simulink model "RL_env"  (R2021b)
settings: Solver=FixedStepAuto  StartTime=0.0  StopTime=Inf  FixedStep=info_.slx_sample_time  RelTol=1e-3
values from neighbouring files (symbols this model uses):
  agent_act_number = 2    [RL_menage.m]
  agent_obs_number = 6    [RL_menage.m]
  agent_sample_time_agent = slx_sample_time    (= 0.1)    [RL_menage.m]
  info_ = info_.add(params_to_save,params_to_save_vals)    [RL_menage.m]
  slx_if_input_normalization = 1    [RL_menage.m]
  slx_if_not_constrain = true    [RL_menage.m]
  slx_multiplier = 1    [RL_menage.m]
  slx_ObsMaximal = repmat(slx_ObsMaximal,1,slx_how_many_steps_in_run)    [RL_menage.m]
  slx_ObsMinimal = zeros(agent_obs_number,1); end    [RL_menage.m]
  slx_sample_time = slx_sample_time_in    (= 0.1)    [RL_menage.m]
  slx_use_external = false    [RL_menage.m]
  slx_w1 = slx_w1_in    (= 1)    [RL_menage.m]
  slx_w2 = slx_w2_in    (= 0)    [RL_menage.m]
undefined symbols (not defined in the file or in its folder): agent_data_random_seed_1, agent_data_random_seed_2, slx_constr_bound, umax
libraries: dspindex x2, rllib x1, simulink x1
settings Model: Creator=krzysztof  LastModifiedBy=Randomowa Nazwa
settings DataIOCC: SignalLogging=off
settings ModelReferenceCC: ModelReferenceNumInstancesAllowed=Single

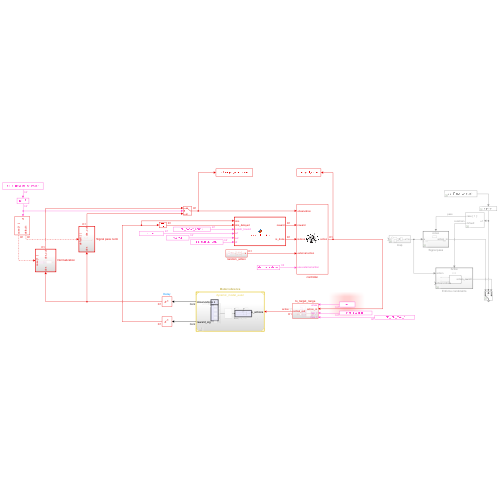
[thumbnail: Simulink's stored preview of the top-level diagram]
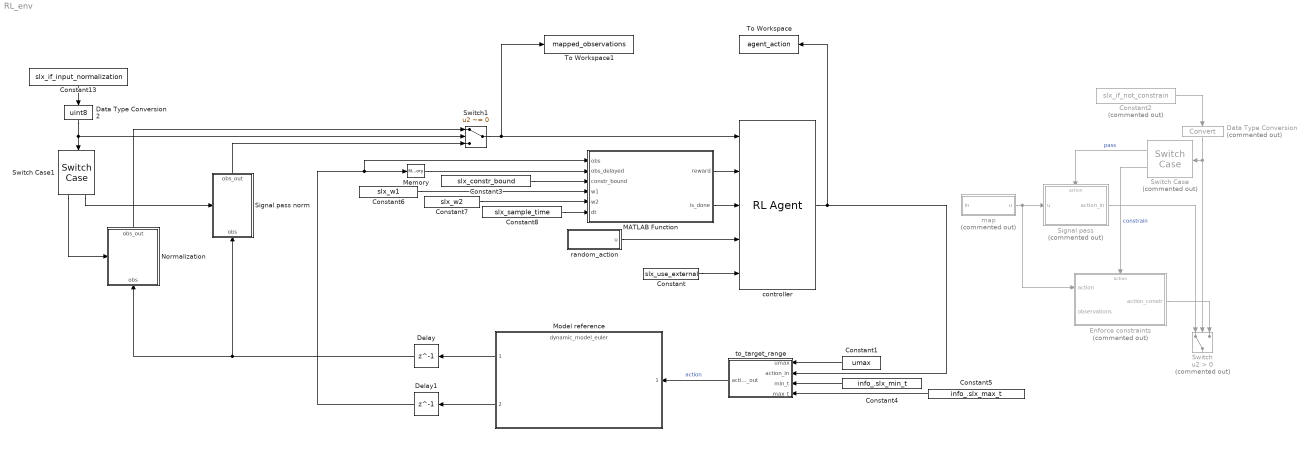
== system RL_env ==
  Constant : Constant  Value=slx_use_external
  Constant1 : Constant  Value=umax
  Constant13 : Constant  Value=slx_if_input_normalization
  Constant2 : Constant  Commented=on  Value=slx_if_not_constrain
  Constant3 : Constant  Value=slx_constr_bound
  Constant4 : Constant  Value=info_.slx_min_t
  Constant5 : Constant  Value=info_.slx_max_t
  Constant6 : Constant  Value=slx_w1
  Constant7 : Constant  Value=slx_w2
  Constant8 : Constant  Value=slx_sample_time
  Data Type Conversion : DataTypeConversion  Commented=on
  Data Type Conversion2 : DataTypeConversion  OutDataTypeStr=uint8
  Delay : Delay  DelayLength=1  InitialCondition=0
  Delay1 : Delay  DelayLength=1  InitialCondition=0
  Enforce constraints : Subsystem  Commented=on  TreatAsAtomicUnit=on
  MATLAB Function : MATLAB Function  TreatAsAtomicUnit=on
  Memory : Memory
  Model reference : ModelReference  ModelNameDialog=dynamic_model_euler.slx  SimulationMode=Normal  ModelReferenceVersion=6.750
  Normalization : Subsystem  TreatAsAtomicUnit=on
  Signal pass : Subsystem  Commented=on  TreatAsAtomicUnit=on
  Signal pass norm : Subsystem  TreatAsAtomicUnit=on
  Switch : Switch  Commented=on  Criteria=u2 > Threshold
  Switch Case : SwitchCase  Commented=on
  Switch Case1 : SwitchCase
  Switch1 : Switch  Criteria=u2 ~= 0
  To Workspace : ToWorkspace  VariableName=agent_action  SaveFormat=Timeseries  SampleTime=-1
  To Workspace1 : ToWorkspace  VariableName=mapped_observations  SaveFormat=Timeseries  SampleTime=-1
  controller : rllib/RL Agent  Agent=agentObj  ExternalActionAsInput=on  ProvideCumRwd=off  TreatAsDirectFeedthrough=on
  map : Subsystem  Commented=on
  random_action : Subsystem
  to_target_range : Subsystem
  wires:
  MATLAB Function/1(reward) -> controller/2
  MATLAB Function/2(is_done) -> controller/3
  Constant/1 -> controller/5
  Constant1/1 -> to_target_range/1(umax)
  Switch Case/2 -> Enforce constraints/Action  "constrain"
  Switch Case/1 -> Signal pass/Action  "pass"
  Signal pass/1(action_in) -> Switch/1
  Enforce constraints/1(action_constr) -> Switch/3
  Constant2/1 -> Data Type Conversion/1
  Data Type Conversion/1 -> Switch/2, Switch Case/1
  Constant3/1 -> MATLAB Function/3(constr_bound)
  random_action/1(u) -> controller/4
  controller/1 -> to_target_range/2(action_in), To Workspace/1
  map/1(u) -> Enforce constraints/1(action), Signal pass/1(u)
  Constant4/1 -> to_target_range/3(min_t)
  Constant5/1 -> to_target_range/4(max_t)
  Constant6/1 -> MATLAB Function/4(w1)
  Constant7/1 -> MATLAB Function/5(w2)
  Model reference/2 -> Delay1/1
  Constant8/1 -> MATLAB Function/6(dt)
  Switch1/1 -> To Workspace1/1, controller/1
  Model reference/1 -> Delay/1
  Memory/1 -> MATLAB Function/2(obs_delayed)
  Constant13/1 -> Data Type Conversion2/1
  Switch Case1/1 -> Normalization/Action
  Switch Case1/2 -> Signal pass norm/Action
  Data Type Conversion2/1 -> Switch1/2, Switch Case1/1
  Signal pass norm/1(obs_out) -> Switch1/3
  Normalization/1(obs_out) -> Switch1/1
  Delay/1 -> Normalization/1(obs), Signal pass norm/1(obs)
  Delay1/1 -> MATLAB Function/1(obs), Memory/1
  to_target_range/1(action_out) -> Model reference/1  "action"

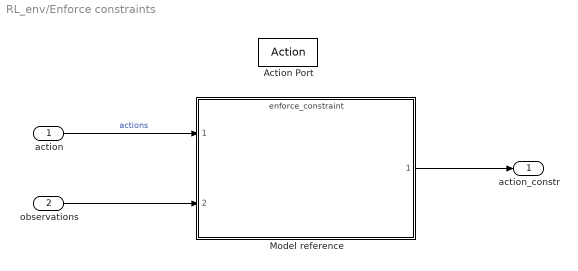
== system RL_env/Enforce constraints ==
  action : Inport  PortDimensions="[agent_act_number  1 ]"
  observations : Inport  Port=2  PortDimensions="[agent_obs_number  1]"
  Action Port : ActionPort
  Model reference : ModelReference  ModelNameDialog=enforce_constraint.slx  SimulationMode=Normal  ModelReferenceVersion=1.89
  action_constr : Outport
  wires:
  action/1 -> Model reference/1  "actions"
  Model reference/1 -> action_constr/1
  observations/1 -> Model reference/2

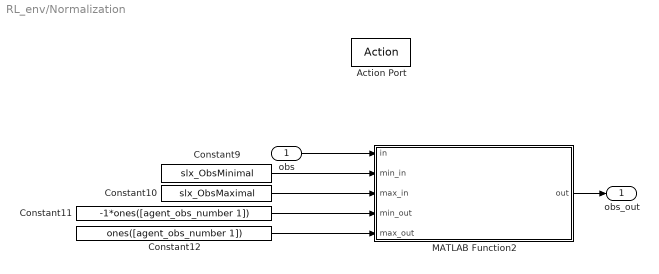
== system RL_env/Normalization ==
  obs : Inport
  Action Port : ActionPort  ActionPortLabel=case [ 1 ]:
  Constant10 : Constant  Value=slx_ObsMaximal
  Constant11 : Constant  Value=-1*ones([agent_obs_number 1])
  Constant12 : Constant  Value=ones([agent_obs_number 1])
  Constant9 : Constant  Value=slx_ObsMinimal
  MATLAB Function2 : MATLAB Function  TreatAsAtomicUnit=on
  obs_out : Outport
  wires:
  Constant9/1 -> MATLAB Function2/2(min_in)
  Constant10/1 -> MATLAB Function2/3(max_in)
  Constant11/1 -> MATLAB Function2/4(min_out)
  Constant12/1 -> MATLAB Function2/5(max_out)
  obs/1 -> MATLAB Function2/1(in)
  MATLAB Function2/1(out) -> obs_out/1

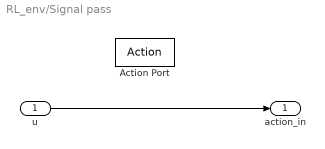
== system RL_env/Signal pass ==
  u : Inport
  Action Port : ActionPort
  action_in : Outport
  wires:
  u/1 -> action_in/1

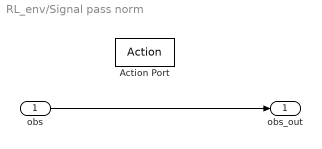
== system RL_env/Signal pass norm ==
  obs : Inport
  Action Port : ActionPort  ActionPortLabel=default:
  obs_out : Outport
  wires:
  obs/1 -> obs_out/1

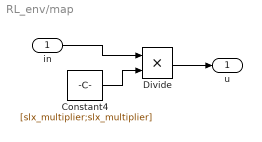
== system RL_env/map ==
  in : Inport
  Constant4 : Constant  Value=[slx_multiplier;slx_multiplier]
  Divide : Product  Inputs=**
  u : Outport
  wires:
  in/1 -> Divide/1
  Constant4/1 -> Divide/2
  Divide/1 -> u/1

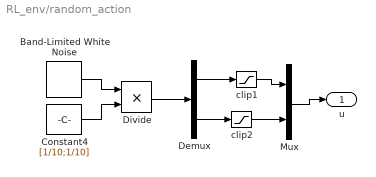
== system RL_env/random_action ==
  Band-Limited White Noise : simulink/Sources/Band-Limited White Noise  Cov=[0.1]  Ts=agent_sample_time_agent  seed=[agent_data_random_seed_1;agent_data_random_seed_2]  VectorParams1D=off
  Constant4 : Constant  Value=[1/10;1/10]
  Demux : Demux  Outputs=2
  Divide : Product  Inputs=**
  Mux : Mux  Inputs=2
  clip1 : Saturate  UpperLimit=1  LowerLimit=-1
  clip2 : Saturate  UpperLimit=1  LowerLimit=-1
  u : Outport
  wires:
  Band-Limited White Noise/1 -> Divide/1
  Constant4/1 -> Divide/2
  Demux/1 -> clip1/1
  clip1/1 -> Mux/1
  Demux/2 -> clip2/1
  clip2/1 -> Mux/2
  Mux/1 -> u/1
  Divide/1 -> Demux/1

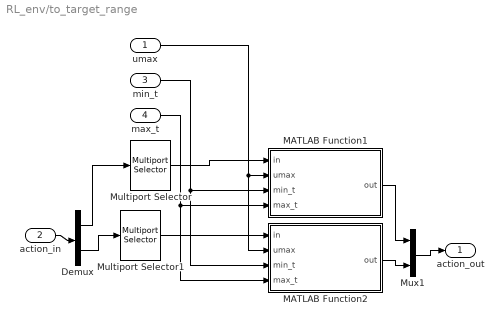
== system RL_env/to_target_range ==
  umax : Inport
  action_in : Inport  Port=2  PortDimensions=[agent_act_number 1 ]
  min_t : Inport  Port=3
  max_t : Inport  Port=4
  Demux : Demux  Outputs=2
  MATLAB Function1 : MATLAB Function  TreatAsAtomicUnit=on
  MATLAB Function2 : MATLAB Function  TreatAsAtomicUnit=on
  Multiport Selector : dspindex/Multiport Selector  rowsOrCols=Rows  idxCellArray={1}  idxErrMode=Clip Index
  Multiport Selector1 : dspindex/Multiport Selector  rowsOrCols=Rows  idxCellArray={1}  idxErrMode=Clip Index
  Mux1 : Mux  Inputs=2
  action_out : Outport  PortDimensions=[agent_act_number 1]
  wires:
  action_in/1 -> Demux/1
  umax/1 -> MATLAB Function2/2(umax), MATLAB Function1/2(umax)
  Demux/2 -> Multiport Selector1/1
  Mux1/1 -> action_out/1
  MATLAB Function1/1(out) -> Mux1/1
  Demux/1 -> Multiport Selector/1
  Multiport Selector/1 -> MATLAB Function1/1(in)
  Multiport Selector1/1 -> MATLAB Function2/1(in)
  MATLAB Function2/1(out) -> Mux1/2
  min_t/1 -> MATLAB Function1/3(min_t), MATLAB Function2/3(min_t)
  max_t/1 -> MATLAB Function2/4(max_t), MATLAB Function1/4(max_t)

== matlab function RL_env/to_target_range/MATLAB Function1 ==
  data: in input; out output; umax input; min_t input; max_t input
function out = mapping(in,umax, min_t, max_t)
    out = [map_m(in(1), min_t, max_t, -umax, umax) ];

== matlab function RL_env/MATLAB Function ==
  data: obs input; obs_delayed input; reward output; is_done output; constr_bound input; w1 input; w2 input; dt input
function [reward, is_done] = reward_function(obs, obs_delayed, constr_bound, w1, w2, dt)

% observations[1] = w_p1
% observations[2] = w_p2
% observations[3] = w_p3
% observations[4] = angle_zb_zw
% global episode_counter;
% episode_counter = episode_counter + 1;

% mean_mag_Hdot = (abs(now(1))+abs(minus1(1))+abs(minus2(3)))/3;
% mean_mag_udot = (abs(now(2))+abs(minus1(2))+abs(minus2(2)))/3;

% reward - minus length of a vector (finds the one with pause before =)
%reward= -sqrt(obs(1)^2 + obs(2)^2 + obs(3)^2);
%if obs(5) == 0, reward= 0; else, reward= - w1* (abs(obs(5)));end %- w2*abs(obs(6));
reward = -w1*abs(obs(1))-w2*abs(obs_delayed-obs(1))/dt;

if false, is_done = 1;% srch_flag
% 'srch_flag' is a phrase for which script reading from slx file searches
% as it takes the first line of the result thi comment must be below
else, is_done = 0; end
end

== matlab function RL_env/to_target_range/MATLAB Function2 ==
  data: in input; out output; umax input; min_t input; max_t input
function out = mapping(in,umax, min_t, max_t)
    out = [map_m(in(1), min_t, max_t, -umax, umax) ];

== matlab function RL_env/Normalization/MATLAB Function2 ==
  data: in input; out output; min_in input; max_in input; min_out input; max_out input
function out = mapping(in, min_in, max_in, min_out, max_out)
    out = map_m(in, min_in, max_in, min_out,max_out );
